simulink library "ControllerLibrary"  (R2016a)
settings: Solver=ode45  StartTime=0.0  StopTime=10.0  RelTol=1e-3
undefined symbols (not defined in the file or in its folder): ControlParams, ControlState, LegHipTorqueLimit, ps3Axes, ps3Buttons, ps3Pov, Ts
libraries: slrtlib x11, vrlib x1, simulink x1
settings Model: Creator=oharib  LastModifiedBy=oharib
settings DataIOCC: LimitDataPoints=on
settings DebuggingCC: AllowSymbolicDim=off

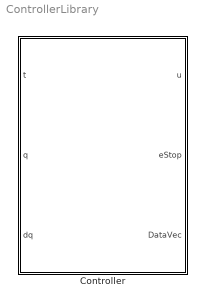
== system ControllerLibrary ==
  Controller : Subsystem

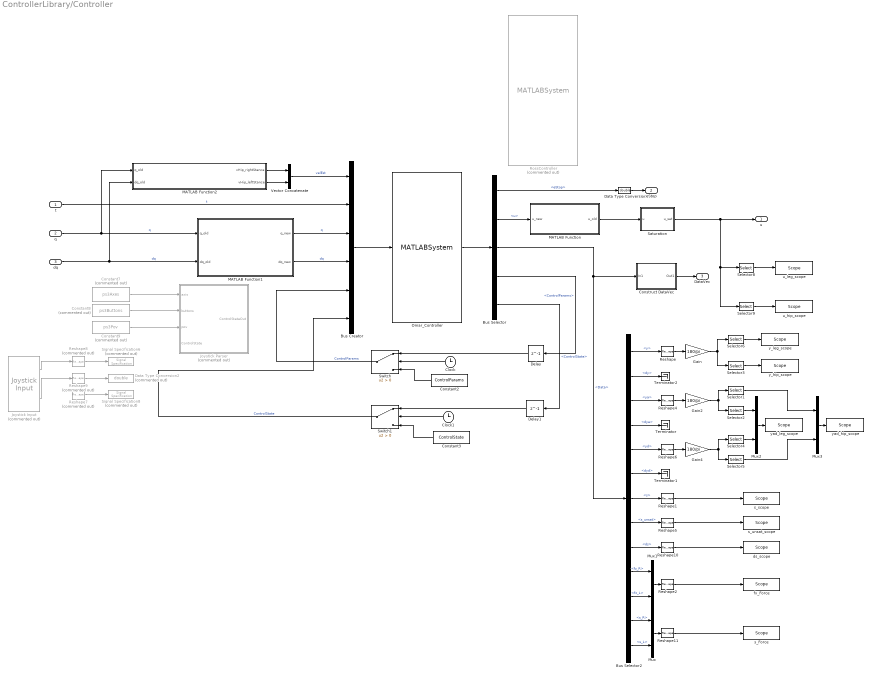
== system ControllerLibrary/Controller ==
  t : Inport
  q : Inport  Port=2
  dq : Inport  Port=3
  Bus Creator : BusCreator  Inputs='velEst','t','q','dq','ControlParams','ControlState'  OutDataTypeStr=Bus: Input_bus
  Bus Selector : BusSelector  OutputSignals=eStop,u,Data,ControlParams,ControlState
  Bus Selector2 : BusSelector  OutputSignals=y,dy,ya,dya,yd,dyd,s,s_unsat,ds,fz_R,fz_L,s_R,s_L
  Clock : Clock
  Clock1 : Clock
  Constant2 : Constant  Value=ControlParams  OutDataTypeStr=Bus: ControlParams_bus
  Constant3 : Constant  Value=ControlState  OutDataTypeStr=Bus: ControlState_bus
  Constant7 : Constant  Commented=on  Value=ps3Axes
  Constant8 : Constant  Commented=on  Value=ps3Buttons
  Constant9 : Constant  Commented=on  Value=ps3Pov
  Construct DataVec : Subsystem
  Data Type Conversion : DataTypeConversion  OutDataTypeStr=double
  Data Type Conversion2 : DataTypeConversion  Commented=on  OutDataTypeStr=double
  Delay : Delay  DelayLength=1  InitialCondition=0  InputProcessing=Inherited
  Delay1 : Delay  DelayLength=1  InitialCondition=0  InputProcessing=Inherited
  Gain : Gain  Gain=180/pi
  Gain2 : Gain  Gain=180/pi
  Gain4 : Gain  Gain=180/pi
  Joystick Input : vrlib/Joystick Input  Commented=on  joyid=1  adjustports=on  forcefeed=off
  Joystick Parser : Subsystem  Commented=on
  MATLAB Function : MATLAB Function  TreatAsAtomicUnit=on
  MATLAB Function1 : MATLAB Function  TreatAsAtomicUnit=on
  MATLAB Function2 : MATLAB Function  TreatAsAtomicUnit=on
  Mux{,1..3} (4 alike) : Mux  Inputs=2
  Omar_Controller : MATLABSystem  System=CompliantController.Omar_Controller  kp=kp_ctrl  kd=kd_ctrl  kp_hip=kp_hip_ctrl  kd_hip=kd_hip_ctrl  hold=hold_ctrl  shakeholdtest=1  controller_choice=controller_choice_ctrl  Ts=Ts  zero_error=zero_error_ctrl  torso_control=torso_control_ctrl  regulate_velocity=regulate_velocity_ctrl  threeD=threeD_ctrl  LimitSwHipAngle=LimitSwHipAngle_ctrl  jointPassivity=jointPassivity_ctrl  footPlacementLA=footPlacementLA_ctrl  footPlacementHA=footPlacementHA_ctrl  s_period=s_period_ctrl  number_of_domains_per_leg=4  deltaStKA=deltaStKA_ctrl  deltaSwKA=deltaSwKA_ctrl  deltaSwLA=deltaSwLA_ctrl  deltaSwHA=deltaSwHA_ctrl  joint_test_link_num=joint_test_link_num_ctrl  joint_test_freq=joint_test_freq_ctrl  joint_test_amp=joint_test_amp_ctrl  joint_zero=joint_zero_ctrl  isSim=isSim  OutputBusName=Output_bus  SimulateUsing=Code generation
      mask Type: CompliantController.Omar_Controller
      mask Display:
      | disp('Omar_Controller');
      | port_label('input',1,'input');
      | port_label('output',1,'output');
  Reshape{,1..2,4..6,10..11} (8 alike) : Reshape
  Reshape7 : Reshape  Commented=on  OutputDimensionality=Row vector (2-D)
  Reshape8 : Reshape  Commented=on  OutputDimensionality=Row vector (2-D)
  Reshape9 : Reshape  Commented=on  OutputDimensionality=Row vector (2-D)
  RossController : MATLABSystem  Commented=on  System=Ross_Controller_obj  kp_pitch=40  kd_pitch=1  kp_roll=40  kd_roll=1  kp_stanceLeg=40  kd_stanceLeg=1  kp_swingLeg=40  kd_swingLeg=1  kp_stanceKnee=40  kd_stanceKnee=1  kp_swingKnee=40  kd_swingKnee=1  kp_stanceHip=40  kd_stanceHip=1  kp_swingHip=40  kd_swingHip=1  tau=0.25  kf_sla=0  kp_sla=0.3  kd_sla=0.1  ki_sla=0  kg_sla=0  kf_sha=0.15  kp_sha=0.1  kd_sha=0.2  ki_sha=0  kg_sha=0  thres_lo=150  thres_hi=250  uHipGravity=0.9  springDeflectionImpactThreshold=0.0262  leg_length=0.6  torso_com_offset=[ 0; 0; 0 ]  isTest_holdInAir=false  isTest_doubleSupport=false  isTest_stopAndGo=false  isTest_constantHips=false  isTest_hipTracking=false  isSim=true  OutputBusName=Output_bus  SimulateUsing=Interpreted execution
      mask Type: Ross_Controller_obj
      mask Display:
      | disp('Ross_Controller_obj');
      | port_label('input',1,'input');
      | port_label('output',1,'output');
  Saturation : Subsystem
  Selector1 : Selector  InputPortWidth=6  IndexOptions=Index vector (dialog)  Indices=[1,4]  OutputSizes=1
  Selector2 : Selector  InputPortWidth=6  IndexOptions=Index vector (dialog)  Indices=[2,3,5,6]  OutputSizes=1
  Selector3 : Selector  InputPortWidth=6  IndexOptions=Index vector (dialog)  Indices=[1, 4]  OutputSizes=1
  Selector4 : Selector  InputPortWidth=6  IndexOptions=Index vector (dialog)  Indices=[2,3,5,6]  OutputSizes=1
  Selector5 : Selector  InputPortWidth=6  IndexOptions=Index vector (dialog)  Indices=[1,4]  OutputSizes=1
  Selector6 : Selector  InputPortWidth=6  IndexOptions=Index vector (dialog)  Indices=[2,3,5,6]  OutputSizes=1
  Selector8 : Selector  InputPortWidth=6  IndexOptions=Index vector (dialog)  Indices=[1, 2, 4, 5]  OutputSizes=1
  Selector9 : Selector  InputPortWidth=6  IndexOptions=Index vector (dialog)  Indices=[3, 6]  OutputSizes=1
  Signal Specification6 : SignalSpecification  Commented=on  OutDataTypeStr=double  Dimensions=5
  Signal Specification8 : SignalSpecification  Commented=on  OutDataTypeStr=double
  Switch : Switch  Criteria=u2 > Threshold
  Switch1 : Switch  Criteria=u2 > Threshold
  Terminator : Terminator
  Terminator1 : Terminator
  Terminator2 : Terminator
  Vector Concatenate : Concatenate
  ds_scope : slrtlib/Displays and Logging/Scope   scopeno=1  scopetype=Host  autostart=on  viewmode=Graphical redraw  formatstr='%15.6f'  grid=on  ylimits=[0,0]  nosamples=2500  noprepostsamples=0  interleave=1  triggermode=FreeRun  triggersignal=1  trigsignalfromport=off  triggerlevel=0.0  triggerslope=Either  triggerscope=1  triggersample=0  filename=data.dat  mode=Lazy  writesize=512  autorestart=off  dynamicfilemode=off  maxwritefilesize=512*1024^2
  fx_Force : slrtlib/Displays and Logging/Scope   scopeno=2  scopetype=Host  autostart=on  viewmode=Graphical redraw  formatstr='%15.6f'  grid=on  ylimits=[0,0]  nosamples=2500  noprepostsamples=0  interleave=1  triggermode=FreeRun  triggersignal=1  trigsignalfromport=off  triggerlevel=0.0  triggerslope=Either  triggerscope=1  triggersample=0  filename=data.dat  mode=Lazy  writesize=512  autorestart=off  dynamicfilemode=off  maxwritefilesize=512*1024^2
  s_Force : slrtlib/Displays and Logging/Scope   scopeno=14  scopetype=Host  autostart=on  viewmode=Graphical redraw  formatstr='%15.6f'  grid=on  ylimits=[0,0]  nosamples=2500  noprepostsamples=0  interleave=1  triggermode=FreeRun  triggersignal=1  trigsignalfromport=off  triggerlevel=0.0  triggerslope=Either  triggerscope=1  triggersample=0  filename=data.dat  mode=Lazy  writesize=512  autorestart=off  dynamicfilemode=off  maxwritefilesize=512*1024^2
  s_scope : slrtlib/Displays and Logging/Scope   scopeno=5  scopetype=Host  autostart=on  viewmode=Graphical redraw  formatstr='%15.6f'  grid=on  ylimits=[0,0]  nosamples=2500  noprepostsamples=0  interleave=1  triggermode=FreeRun  triggersignal=1  trigsignalfromport=off  triggerlevel=0.0  triggerslope=Either  triggerscope=1  triggersample=0  filename=data.dat  mode=Lazy  writesize=512  autorestart=off  dynamicfilemode=off  maxwritefilesize=512*1024^2
  s_unsat_scope : slrtlib/Displays and Logging/Scope   scopeno=6  scopetype=Host  autostart=on  viewmode=Graphical redraw  formatstr='%15.6f'  grid=on  ylimits=[0,0]  nosamples=2500  noprepostsamples=0  interleave=1  triggermode=FreeRun  triggersignal=1  trigsignalfromport=off  triggerlevel=0.0  triggerslope=Either  triggerscope=1  triggersample=0  filename=data.dat  mode=Lazy  writesize=512  autorestart=off  dynamicfilemode=off  maxwritefilesize=512*1024^2
  u_hip_scope : slrtlib/Displays and Logging/Scope   scopeno=8  scopetype=Host  autostart=on  viewmode=Graphical redraw  formatstr='%15.6f'  grid=on  ylimits=[0,0]  nosamples=2500  noprepostsamples=0  interleave=1  triggermode=FreeRun  triggersignal=1  trigsignalfromport=off  triggerlevel=0.0  triggerslope=Either  triggerscope=1  triggersample=0  filename=data.dat  mode=Lazy  writesize=512  autorestart=off  dynamicfilemode=off  maxwritefilesize=512*1024^2
  u_leg_scope : slrtlib/Displays and Logging/Scope   scopeno=7  scopetype=Host  autostart=on  viewmode=Graphical redraw  formatstr='%15.6f'  grid=on  ylimits=[0,0]  nosamples=2500  noprepostsamples=0  interleave=1  triggermode=FreeRun  triggersignal=1  trigsignalfromport=off  triggerlevel=0.0  triggerslope=Either  triggerscope=1  triggersample=0  filename=data.dat  mode=Lazy  writesize=512  autorestart=off  dynamicfilemode=off  maxwritefilesize=512*1024^2
  y_hip_scope : slrtlib/Displays and Logging/Scope   scopeno=9  scopetype=Host  autostart=on  viewmode=Graphical redraw  formatstr='%15.6f'  grid=on  ylimits=[0,0]  nosamples=2500  noprepostsamples=0  interleave=1  triggermode=FreeRun  triggersignal=1  trigsignalfromport=off  triggerlevel=0.0  triggerslope=Either  triggerscope=1  triggersample=0  filename=data.dat  mode=Lazy  writesize=512  autorestart=off  dynamicfilemode=off  maxwritefilesize=512*1024^2
  y_leg_scope : slrtlib/Displays and Logging/Scope   scopeno=4  scopetype=Host  autostart=on  viewmode=Graphical redraw  formatstr='%15.6f'  grid=on  ylimits=[0,0]  nosamples=2500  noprepostsamples=0  interleave=1  triggermode=FreeRun  triggersignal=1  trigsignalfromport=off  triggerlevel=0.0  triggerslope=Either  triggerscope=1  triggersample=0  filename=data.dat  mode=Lazy  writesize=512  autorestart=off  dynamicfilemode=off  maxwritefilesize=512*1024^2
  yad_hip_scope : slrtlib/Displays and Logging/Scope   scopeno=10  scopetype=Host  autostart=on  viewmode=Graphical redraw  formatstr='%15.6f'  grid=on  ylimits=[0,0]  nosamples=2500  noprepostsamples=0  interleave=1  triggermode=FreeRun  triggersignal=1  trigsignalfromport=off  triggerlevel=0.0  triggerslope=Either  triggerscope=1  triggersample=0  filename=data.dat  mode=Lazy  writesize=512  autorestart=off  dynamicfilemode=off  maxwritefilesize=512*1024^2
  yad_leg_scope : slrtlib/Displays and Logging/Scope   scopeno=3  scopetype=Host  autostart=on  viewmode=Graphical redraw  formatstr='%15.6f'  grid=on  ylimits=[0,0]  nosamples=2500  noprepostsamples=0  interleave=1  triggermode=FreeRun  triggersignal=1  trigsignalfromport=off  triggerlevel=0.0  triggerslope=Either  triggerscope=1  triggersample=0  filename=data.dat  mode=Lazy  writesize=512  autorestart=off  dynamicfilemode=off  maxwritefilesize=512*1024^2
  u : Outport  OutDataTypeStr=double
  eStop : Outport  Port=2  OutDataTypeStr=double
  DataVec : Outport  Port=3
  wires:
  dq/1 -> MATLAB Function2/2(dq_old), MATLAB Function1/2(dq_old)  "dq"
  Bus Selector/1 -> Data Type Conversion/1  "<eStop>"
  Data Type Conversion/1 -> eStop/1
  Saturation/1(u_sat) -> u/1, Selector8/1, Selector9/1
  t/1 -> Bus Creator/2  "t"
  Bus Creator/1 -> Omar_Controller/1
  Omar_Controller/1 -> Bus Selector/1
  Bus Selector/3 -> Bus Selector2/1, Construct DataVec/1(In1)  "<Data>"
  Bus Selector/4 -> Delay/1  "<ControlParams>"
  Bus Selector/5 -> Delay1/1  "<ControlState>"
  Delay/1 -> Switch/1
  Delay1/1 -> Switch1/1
  Clock/1 -> Switch/2
  Constant2/1 -> Switch/3
  Clock1/1 -> Switch1/2
  Constant3/1 -> Switch1/3
  Switch1/1 -> Bus Creator/6  "ControlState"
  Joystick Input/2 -> Reshape9/1
  Reshape8/1 -> Signal Specification6/1
  Joystick Input/1 -> Reshape8/1
  Reshape7/1 -> Signal Specification8/1
  Reshape9/1 -> Data Type Conversion2/1
  Construct DataVec/1(Out1) -> DataVec/1
  Constant7/1 -> Joystick Parser/1(axis)
  Constant8/1 -> Joystick Parser/2(buttons)
  q/1 -> MATLAB Function2/1(q_old), MATLAB Function1/1(q_old)  "q"
  MATLAB Function1/1(q_new) -> Bus Creator/3  "q"
  MATLAB Function/1(u_old) -> Saturation/1(u)
  Bus Selector/2 -> MATLAB Function/1(u_new)  "<u>"
  MATLAB Function1/2(dq_new) -> Bus Creator/4  "dq"
  Selector8/1 -> u_leg_scope/1
  Selector9/1 -> u_hip_scope/1
  Bus Selector2/1 -> Reshape/1  "<y>"
  Constant9/1 -> Joystick Parser/3(pov)
  Reshape/1 -> Gain/1
  Reshape4/1 -> Gain2/1
  Reshape6/1 -> Gain4/1
  Bus Selector2/5 -> Reshape6/1  "<yd>"
  Bus Selector2/3 -> Reshape4/1  "<ya>"
  Gain/1 -> Selector3/1, Selector6/1
  Selector3/1 -> y_hip_scope/1
  Bus Selector2/4 -> Terminator/1  "<dya>"
  Bus Selector2/6 -> Terminator1/1  "<dyd>"
  Bus Selector2/2 -> Terminator2/1  "<dy>"
  MATLAB Function2/1(vHip_rightStance) -> Vector Concatenate/1
  MATLAB Function2/2(vHip_leftStance) -> Vector Concatenate/2
  Vector Concatenate/1 -> Bus Creator/1  "velEst"
  Bus Selector2/9 -> Reshape10/1  "<ds>"
  Reshape10/1 -> ds_scope/1
  Reshape5/1 -> s_unsat_scope/1
  Reshape1/1 -> s_scope/1
  Bus Selector2/7 -> Reshape1/1  "<s>"
  Bus Selector2/8 -> Reshape5/1  "<s_unsat>"
  Reshape11/1 -> s_Force/1
  Bus Selector2/12 -> Mux/1  "<s_R>"
  Bus Selector2/13 -> Mux/2  "<s_L>"
  Mux/1 -> Reshape11/1
  Reshape2/1 -> fx_Force/1
  Bus Selector2/10 -> Mux1/1  "<fz_R>"
  Bus Selector2/11 -> Mux1/2  "<fz_L>"
  Mux1/1 -> Reshape2/1
  Gain2/1 -> Selector1/1, Selector2/1
  Gain4/1 -> Selector5/1, Selector4/1
  Selector6/1 -> y_leg_scope/1
  Mux2/1 -> yad_leg_scope/1
  Selector2/1 -> Mux2/1
  Selector4/1 -> Mux2/2
  Mux3/1 -> yad_hip_scope/1
  Selector1/1 -> Mux3/1
  Selector5/1 -> Mux3/2
  Switch/1 -> Bus Creator/5  "ControlParams"

== system ControllerLibrary/Controller/Construct DataVec ==
  In1 : Inport
  DataBusSelector : BusSelector  OutputSignals=q,u,y,dy,ya,dya,yd,dyd,s,s_unsat,ds,Domain,s_R,s_L,fz_R,fz_L,velFiltered,velMeasured,swingHipAdjustment,swingLegAdjustment
  DataVectorize : Concatenate  NumInputs=20
  Out1 : Outport
  wires:
  In1/1 -> DataBusSelector/1
  DataVectorize/1 -> Out1/1
  DataBusSelector/1 -> DataVectorize/1  "<q>"
  DataBusSelector/2 -> DataVectorize/2  "<u>"
  DataBusSelector/3 -> DataVectorize/3  "<y>"
  DataBusSelector/4 -> DataVectorize/4  "<dy>"
  DataBusSelector/5 -> DataVectorize/5  "<ya>"
  DataBusSelector/6 -> DataVectorize/6  "<dya>"
  DataBusSelector/7 -> DataVectorize/7  "<yd>"
  DataBusSelector/8 -> DataVectorize/8  "<dyd>"
  DataBusSelector/9 -> DataVectorize/9  "<s>"
  DataBusSelector/10 -> DataVectorize/10  "<s_unsat>"
  DataBusSelector/11 -> DataVectorize/11  "<ds>"
  DataBusSelector/12 -> DataVectorize/12  "<Domain>"
  DataBusSelector/13 -> DataVectorize/13  "<s_R>"
  DataBusSelector/14 -> DataVectorize/14  "<s_L>"
  DataBusSelector/15 -> DataVectorize/15  "<fz_R>"
  DataBusSelector/16 -> DataVectorize/16  "<fz_L>"
  DataBusSelector/17 -> DataVectorize/17  "<velFiltered>"
  DataBusSelector/18 -> DataVectorize/18  "<velMeasured>"
  DataBusSelector/19 -> DataVectorize/19  "<swingHipAdjustment>"
  DataBusSelector/20 -> DataVectorize/20  "<swingLegAdjustment>"

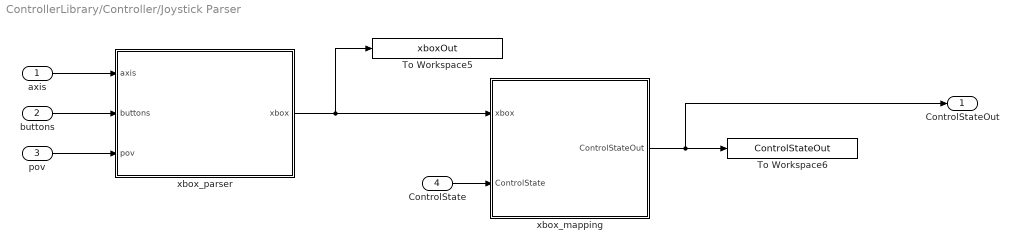
== system ControllerLibrary/Controller/Joystick Parser ==
  axis : Inport
  buttons : Inport  Port=2
  pov : Inport  Port=3
  ControlState : Inport  Port=4  OutDataTypeStr=Bus: ControlState_bus
  To Workspace5 : ToWorkspace  VariableName=xboxOut  SaveFormat=Timeseries  SampleTime=-1
  To Workspace6 : ToWorkspace  VariableName=ControlStateOut  SaveFormat=Timeseries  SampleTime=-1
  xbox_mapping : Subsystem
  xbox_parser : MATLAB Function  TreatAsAtomicUnit=on
  ControlStateOut : Outport  OutDataTypeStr=Bus: ControlState_bus
  wires:
  xbox_parser/1(xbox) -> To Workspace5/1, xbox_mapping/1(xbox)
  xbox_mapping/1(ControlStateOut) -> To Workspace6/1, ControlStateOut/1
  axis/1 -> xbox_parser/1(axis)
  buttons/1 -> xbox_parser/2(buttons)
  pov/1 -> xbox_parser/3(pov)
  ControlState/1 -> xbox_mapping/2(ControlState)

== system ControllerLibrary/Controller/Saturation ==
  u : Inport
  Data Type Conversion1 : DataTypeConversion  OutDataTypeStr=double
  Gain : Gain  Gain=-1
  Gain1 : Gain  Gain=[1 0; 1 0; 0 1; 1 0; 1 0; 0 1]  Multiplication=Matrix(K*u)
  LegHipTorqueSat : Constant  Value=LegHipTorqueLimit
  Saturation Dynamic : simulink/Discontinuities/Saturation Dynamic  OutMin=[]  OutMax=[]  OutDataTypeStr=Inherit: Same as second input  OutDataType=fixdt(1, 16)  OutScaling=2^-10  DoSatur=off
  u_sat : Outport  OutDataTypeStr=double
  wires:
  Saturation Dynamic/1 -> Data Type Conversion1/1
  Data Type Conversion1/1 -> u_sat/1  "torque_sat"
  LegHipTorqueSat/1 -> Gain1/1
  Gain1/1 -> Saturation Dynamic/1, Gain/1
  Gain/1 -> Saturation Dynamic/3
  u/1 -> Saturation Dynamic/2

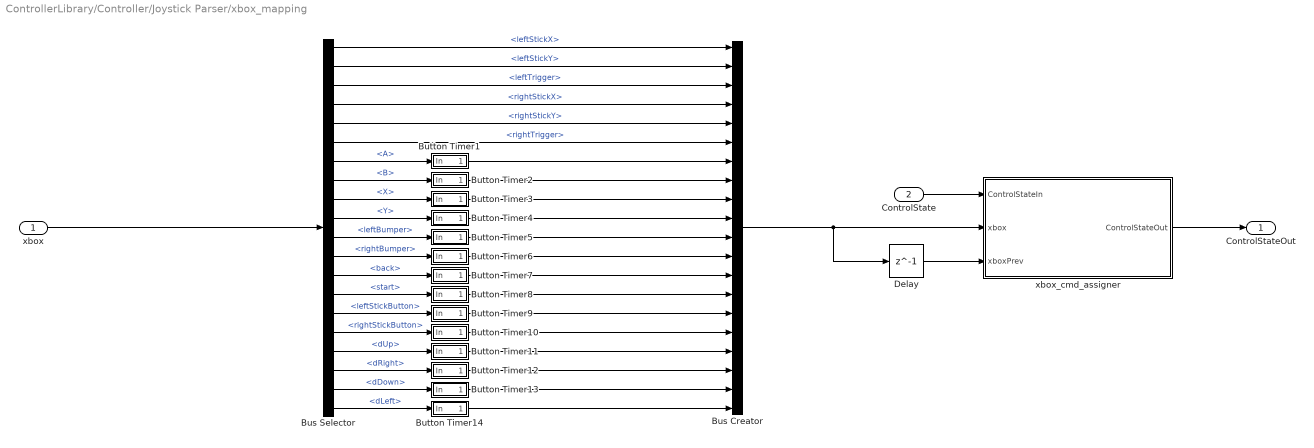
== system ControllerLibrary/Controller/Joystick Parser/xbox_mapping ==
  xbox : Inport
  ControlState : Inport  Port=2  OutDataTypeStr=Bus: ControlState_bus
  Bus Creator : BusCreator  Inputs=20  OutDataTypeStr=Bus: xbox_bus  NonVirtualBus=on
  Bus Selector : BusSelector  OutputSignals=leftStickX,leftStickY,leftTrigger,rightStickX,rightStickY,rightTrigger,A,B,X,Y,leftBumper,rightBumper,back,start,leftStickButton,rightStickButton,dUp,dRight,dDown,dLeft
  Button Timer1 : Subsystem
  Button Timer10 : Subsystem
  Button Timer11 : Subsystem
  Button Timer12 : Subsystem
  Button Timer13 : Subsystem
  Button Timer14 : Subsystem
  Button Timer2 : Subsystem
  Button Timer3 : Subsystem
  Button Timer4 : Subsystem
  Button Timer5 : Subsystem
  Button Timer6 : Subsystem
  Button Timer7 : Subsystem
  Button Timer8 : Subsystem
  Button Timer9 : Subsystem
  Delay : Delay  DelayLength=1  InitialCondition=0
  xbox_cmd_assigner : MATLAB Function  TreatAsAtomicUnit=on
  ControlStateOut : Outport  OutDataTypeStr=Bus: ControlState_bus
  wires:
  Bus Selector/12 -> Button Timer6/1(In)  "<rightBumper>"
  Bus Selector/4 -> Bus Creator/4  "<rightStickX>"
  Bus Selector/3 -> Bus Creator/3  "<leftTrigger>"
  Bus Selector/9 -> Button Timer3/1(In)  "<X>"
  Bus Selector/1 -> Bus Creator/1  "<leftStickX>"
  Bus Selector/5 -> Bus Creator/5  "<rightStickY>"
  Bus Selector/14 -> Button Timer8/1(In)  "<start>"
  Bus Selector/17 -> Button Timer11/1(In)  "<dUp>"
  Bus Selector/18 -> Button Timer12/1(In)  "<dRight>"
  Bus Selector/8 -> Button Timer2/1(In)  "<B>"
  Bus Selector/19 -> Button Timer13/1(In)  "<dDown>"
  Bus Selector/7 -> Button Timer1/1(In)  "<A>"
  Bus Selector/15 -> Button Timer9/1(In)  "<leftStickButton>"
  xbox/1 -> Bus Selector/1
  Bus Selector/6 -> Bus Creator/6  "<rightTrigger>"
  Bus Selector/20 -> Button Timer14/1(In)  "<dLeft>"
  Bus Selector/2 -> Bus Creator/2  "<leftStickY>"
  Bus Selector/10 -> Button Timer4/1(In)  "<Y>"
  Bus Selector/13 -> Button Timer7/1(In)  "<back>"
  Bus Selector/16 -> Button Timer10/1(In)  "<rightStickButton>"
  Bus Selector/11 -> Button Timer5/1(In)  "<leftBumper>"
  Button Timer2/1(Out) -> Bus Creator/8
  Button Timer4/1(Out) -> Bus Creator/10
  Button Timer5/1(Out) -> Bus Creator/11
  Button Timer6/1(Out) -> Bus Creator/12
  Button Timer7/1(Out) -> Bus Creator/13
  Button Timer8/1(Out) -> Bus Creator/14
  Button Timer9/1(Out) -> Bus Creator/15
  Button Timer10/1(Out) -> Bus Creator/16
  Button Timer11/1(Out) -> Bus Creator/17
  Button Timer12/1(Out) -> Bus Creator/18
  Button Timer13/1(Out) -> Bus Creator/19
  Button Timer14/1(Out) -> Bus Creator/20
  Bus Creator/1 -> Delay/1, xbox_cmd_assigner/2(xbox)
  ControlState/1 -> xbox_cmd_assigner/1(ControlStateIn)
  Button Timer1/1(Out) -> Bus Creator/7
  Button Timer3/1(Out) -> Bus Creator/9
  xbox_cmd_assigner/1(ControlStateOut) -> ControlStateOut/1
  Delay/1 -> xbox_cmd_assigner/3(xboxPrev)

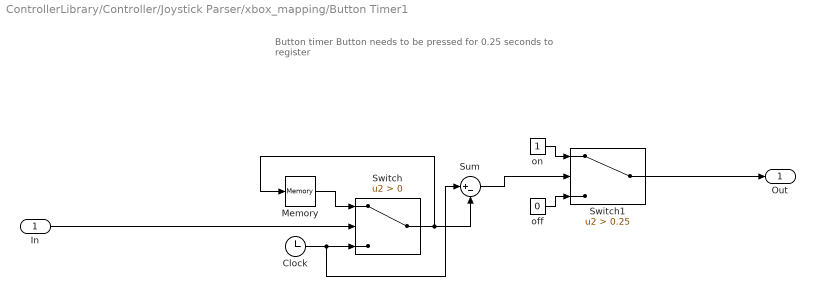
== system ControllerLibrary/Controller/Joystick Parser/xbox_mapping/Button Timer1 ==
  note: Button timer
      | Button needs to be pressed for 0.25 seconds to register
  In : Inport
  Clock : Clock
  Memory : Memory
  Sum : Sum  Inputs=|+-
  Switch : Switch  Criteria=u2 > Threshold
  Switch1 : Switch  Criteria=u2 > Threshold  Threshold=0.25
  off : Constant  Value=0
  on : Constant
  Out : Outport
  wires:
  off/1 -> Switch1/3
  Sum/1 -> Switch1/2
  Switch1/1 -> Out/1
  on/1 -> Switch1/1
  In/1 -> Switch/2
  Clock/1 -> Sum/1, Switch/3
  Memory/1 -> Switch/1
  Switch/1 -> Sum/2, Memory/1

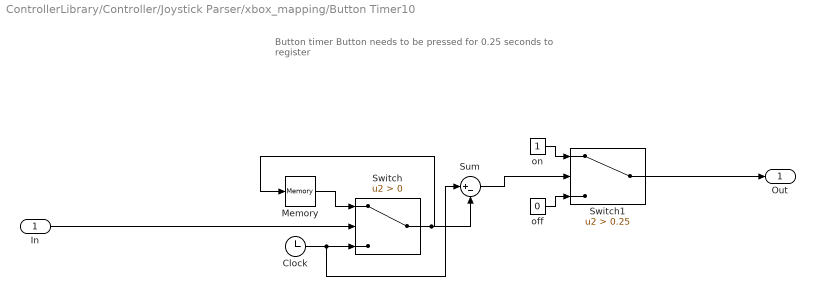
== system ControllerLibrary/Controller/Joystick Parser/xbox_mapping/Button Timer10 ==
  note: Button timer
      | Button needs to be pressed for 0.25 seconds to register
  In : Inport
  Clock : Clock
  Memory : Memory
  Sum : Sum  Inputs=|+-
  Switch : Switch  Criteria=u2 > Threshold
  Switch1 : Switch  Criteria=u2 > Threshold  Threshold=0.25
  off : Constant  Value=0
  on : Constant
  Out : Outport
  wires:
  off/1 -> Switch1/3
  Sum/1 -> Switch1/2
  Switch1/1 -> Out/1
  on/1 -> Switch1/1
  In/1 -> Switch/2
  Clock/1 -> Sum/1, Switch/3
  Memory/1 -> Switch/1
  Switch/1 -> Sum/2, Memory/1

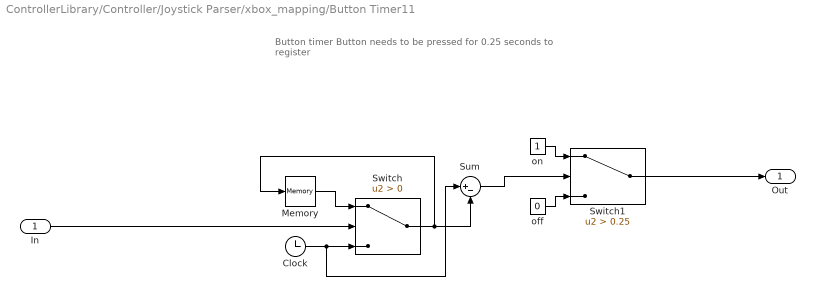
== system ControllerLibrary/Controller/Joystick Parser/xbox_mapping/Button Timer11 ==
  note: Button timer
      | Button needs to be pressed for 0.25 seconds to register
  In : Inport
  Clock : Clock
  Memory : Memory
  Sum : Sum  Inputs=|+-
  Switch : Switch  Criteria=u2 > Threshold
  Switch1 : Switch  Criteria=u2 > Threshold  Threshold=0.25
  off : Constant  Value=0
  on : Constant
  Out : Outport
  wires:
  off/1 -> Switch1/3
  Sum/1 -> Switch1/2
  Switch1/1 -> Out/1
  on/1 -> Switch1/1
  In/1 -> Switch/2
  Clock/1 -> Sum/1, Switch/3
  Memory/1 -> Switch/1
  Switch/1 -> Sum/2, Memory/1

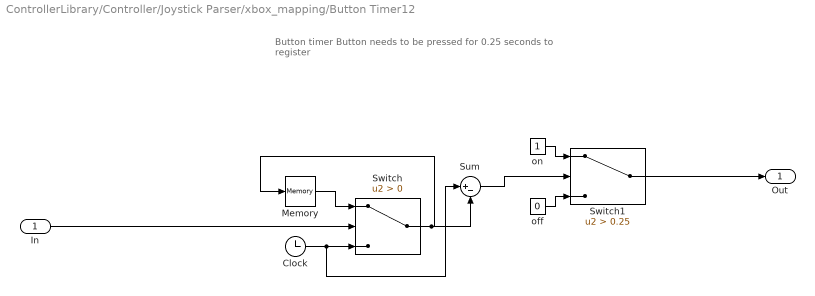
== system ControllerLibrary/Controller/Joystick Parser/xbox_mapping/Button Timer12 ==
  note: Button timer
      | Button needs to be pressed for 0.25 seconds to register
  In : Inport
  Clock : Clock
  Memory : Memory
  Sum : Sum  Inputs=|+-
  Switch : Switch  Criteria=u2 > Threshold
  Switch1 : Switch  Criteria=u2 > Threshold  Threshold=0.25
  off : Constant  Value=0
  on : Constant
  Out : Outport
  wires:
  off/1 -> Switch1/3
  Sum/1 -> Switch1/2
  Switch1/1 -> Out/1
  on/1 -> Switch1/1
  In/1 -> Switch/2
  Clock/1 -> Sum/1, Switch/3
  Memory/1 -> Switch/1
  Switch/1 -> Sum/2, Memory/1

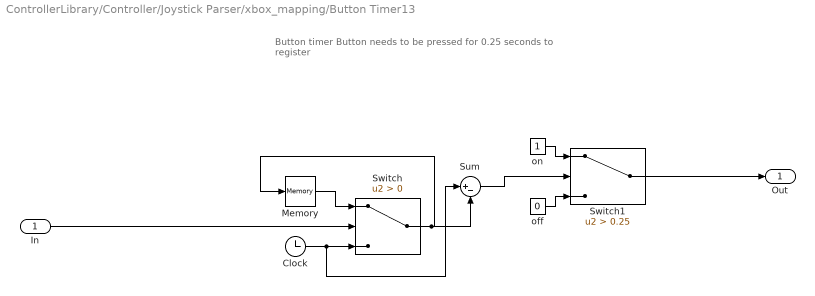
== system ControllerLibrary/Controller/Joystick Parser/xbox_mapping/Button Timer13 ==
  note: Button timer
      | Button needs to be pressed for 0.25 seconds to register
  In : Inport
  Clock : Clock
  Memory : Memory
  Sum : Sum  Inputs=|+-
  Switch : Switch  Criteria=u2 > Threshold
  Switch1 : Switch  Criteria=u2 > Threshold  Threshold=0.25
  off : Constant  Value=0
  on : Constant
  Out : Outport
  wires:
  off/1 -> Switch1/3
  Sum/1 -> Switch1/2
  Switch1/1 -> Out/1
  on/1 -> Switch1/1
  In/1 -> Switch/2
  Clock/1 -> Sum/1, Switch/3
  Memory/1 -> Switch/1
  Switch/1 -> Sum/2, Memory/1

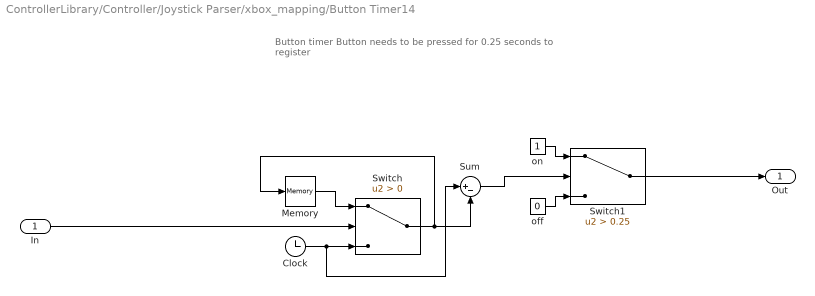
== system ControllerLibrary/Controller/Joystick Parser/xbox_mapping/Button Timer14 ==
  note: Button timer
      | Button needs to be pressed for 0.25 seconds to register
  In : Inport
  Clock : Clock
  Memory : Memory
  Sum : Sum  Inputs=|+-
  Switch : Switch  Criteria=u2 > Threshold
  Switch1 : Switch  Criteria=u2 > Threshold  Threshold=0.25
  off : Constant  Value=0
  on : Constant
  Out : Outport
  wires:
  off/1 -> Switch1/3
  Sum/1 -> Switch1/2
  Switch1/1 -> Out/1
  on/1 -> Switch1/1
  In/1 -> Switch/2
  Clock/1 -> Sum/1, Switch/3
  Memory/1 -> Switch/1
  Switch/1 -> Sum/2, Memory/1

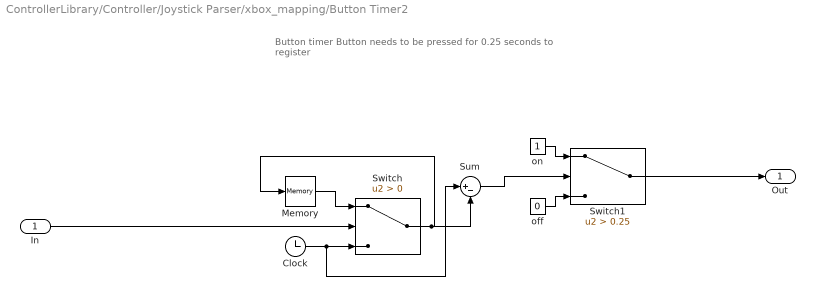
== system ControllerLibrary/Controller/Joystick Parser/xbox_mapping/Button Timer2 ==
  note: Button timer
      | Button needs to be pressed for 0.25 seconds to register
  In : Inport
  Clock : Clock
  Memory : Memory
  Sum : Sum  Inputs=|+-
  Switch : Switch  Criteria=u2 > Threshold
  Switch1 : Switch  Criteria=u2 > Threshold  Threshold=0.25
  off : Constant  Value=0
  on : Constant
  Out : Outport
  wires:
  off/1 -> Switch1/3
  Sum/1 -> Switch1/2
  Switch1/1 -> Out/1
  on/1 -> Switch1/1
  In/1 -> Switch/2
  Clock/1 -> Sum/1, Switch/3
  Memory/1 -> Switch/1
  Switch/1 -> Sum/2, Memory/1

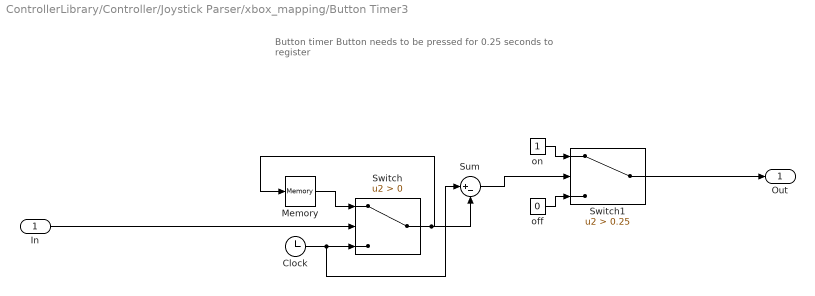
== system ControllerLibrary/Controller/Joystick Parser/xbox_mapping/Button Timer3 ==
  note: Button timer
      | Button needs to be pressed for 0.25 seconds to register
  In : Inport
  Clock : Clock
  Memory : Memory
  Sum : Sum  Inputs=|+-
  Switch : Switch  Criteria=u2 > Threshold
  Switch1 : Switch  Criteria=u2 > Threshold  Threshold=0.25
  off : Constant  Value=0
  on : Constant
  Out : Outport
  wires:
  off/1 -> Switch1/3
  Sum/1 -> Switch1/2
  Switch1/1 -> Out/1
  on/1 -> Switch1/1
  In/1 -> Switch/2
  Clock/1 -> Sum/1, Switch/3
  Memory/1 -> Switch/1
  Switch/1 -> Sum/2, Memory/1

== system ControllerLibrary/Controller/Joystick Parser/xbox_mapping/Button Timer4 ==
  note: Button timer
      | Button needs to be pressed for 0.25 seconds to register
  In : Inport
  Clock : Clock
  Memory : Memory
  Sum : Sum  Inputs=|+-
  Switch : Switch  Criteria=u2 > Threshold
  Switch1 : Switch  Criteria=u2 > Threshold  Threshold=0.25
  off : Constant  Value=0
  on : Constant
  Out : Outport
  wires:
  off/1 -> Switch1/3
  Sum/1 -> Switch1/2
  Switch1/1 -> Out/1
  on/1 -> Switch1/1
  In/1 -> Switch/2
  Clock/1 -> Sum/1, Switch/3
  Memory/1 -> Switch/1
  Switch/1 -> Sum/2, Memory/1

== system ControllerLibrary/Controller/Joystick Parser/xbox_mapping/Button Timer5 ==
  note: Button timer
      | Button needs to be pressed for 0.25 seconds to register
  In : Inport
  Clock : Clock
  Memory : Memory
  Sum : Sum  Inputs=|+-
  Switch : Switch  Criteria=u2 > Threshold
  Switch1 : Switch  Criteria=u2 > Threshold  Threshold=0.25
  off : Constant  Value=0
  on : Constant
  Out : Outport
  wires:
  off/1 -> Switch1/3
  Sum/1 -> Switch1/2
  Switch1/1 -> Out/1
  on/1 -> Switch1/1
  In/1 -> Switch/2
  Clock/1 -> Sum/1, Switch/3
  Memory/1 -> Switch/1
  Switch/1 -> Sum/2, Memory/1

== system ControllerLibrary/Controller/Joystick Parser/xbox_mapping/Button Timer6 ==
  note: Button timer
      | Button needs to be pressed for 0.25 seconds to register
  In : Inport
  Clock : Clock
  Memory : Memory
  Sum : Sum  Inputs=|+-
  Switch : Switch  Criteria=u2 > Threshold
  Switch1 : Switch  Criteria=u2 > Threshold  Threshold=0.25
  off : Constant  Value=0
  on : Constant
  Out : Outport
  wires:
  off/1 -> Switch1/3
  Sum/1 -> Switch1/2
  Switch1/1 -> Out/1
  on/1 -> Switch1/1
  In/1 -> Switch/2
  Clock/1 -> Sum/1, Switch/3
  Memory/1 -> Switch/1
  Switch/1 -> Sum/2, Memory/1

== system ControllerLibrary/Controller/Joystick Parser/xbox_mapping/Button Timer7 ==
  note: Button timer
      | Button needs to be pressed for 0.25 seconds to register
  In : Inport
  Clock : Clock
  Memory : Memory
  Sum : Sum  Inputs=|+-
  Switch : Switch  Criteria=u2 > Threshold
  Switch1 : Switch  Criteria=u2 > Threshold  Threshold=0.25
  off : Constant  Value=0
  on : Constant
  Out : Outport
  wires:
  off/1 -> Switch1/3
  Sum/1 -> Switch1/2
  Switch1/1 -> Out/1
  on/1 -> Switch1/1
  In/1 -> Switch/2
  Clock/1 -> Sum/1, Switch/3
  Memory/1 -> Switch/1
  Switch/1 -> Sum/2, Memory/1

== system ControllerLibrary/Controller/Joystick Parser/xbox_mapping/Button Timer8 ==
  note: Button timer
      | Button needs to be pressed for 0.25 seconds to register
  In : Inport
  Clock : Clock
  Memory : Memory
  Sum : Sum  Inputs=|+-
  Switch : Switch  Criteria=u2 > Threshold
  Switch1 : Switch  Criteria=u2 > Threshold  Threshold=0.25
  off : Constant  Value=0
  on : Constant
  Out : Outport
  wires:
  off/1 -> Switch1/3
  Sum/1 -> Switch1/2
  Switch1/1 -> Out/1
  on/1 -> Switch1/1
  In/1 -> Switch/2
  Clock/1 -> Sum/1, Switch/3
  Memory/1 -> Switch/1
  Switch/1 -> Sum/2, Memory/1

== system ControllerLibrary/Controller/Joystick Parser/xbox_mapping/Button Timer9 ==
  note: Button timer
      | Button needs to be pressed for 0.25 seconds to register
  In : Inport
  Clock : Clock
  Memory : Memory
  Sum : Sum  Inputs=|+-
  Switch : Switch  Criteria=u2 > Threshold
  Switch1 : Switch  Criteria=u2 > Threshold  Threshold=0.25
  off : Constant  Value=0
  on : Constant
  Out : Outport
  wires:
  off/1 -> Switch1/3
  Sum/1 -> Switch1/2
  Switch1/1 -> Out/1
  on/1 -> Switch1/1
  In/1 -> Switch/2
  Clock/1 -> Sum/1, Switch/3
  Memory/1 -> Switch/1
  Switch/1 -> Sum/2, Memory/1

== matlab function ControllerLibrary/Controller/MATLAB Function ==
  data: u_new input; u_old output
function u_old = Convert_u_to_old_coordinates(u_new)
%#codegen

% u_new = [qHR, qAR, qBR, qHL, qAL, qBL]
% u_old = [qAR, qBR, qHR, qAL, qBL, qHL]

u_old = u_new([2,3,1,5,6,4]);
u_old(6) = -u_old(6); % Flip left hip torque

end

== matlab function ControllerLibrary/Controller/MATLAB Function1 ==
  data: q_old input; q_new output; dq_old input; dq_new output
function [q_new, dq_new] = Convert_x_to_new_coordinates(q_old, dq_old)
%#codegen
[q_new, dq_new] = CompliantSystem.ConvertToNewCoord(q_old, dq_old);
end

== matlab function ControllerLibrary/Controller/Joystick Parser/xbox_mapping/xbox_cmd_assigner ==
  data: ControlStateIn input; xbox input; ControlStateOut output Bus: ControlState_bus; xboxPrev input
function ControlStateOut = xbox_cmd_assigner(ControlStateIn, xbox, xboxPrev) %#codegen
%% Copyright 2016 - Ross Hartley

ControlStateOut = ControlStateIn;
sampleInterval = 0.0005;

%% Commands 

% Shutdown
if xbox.back == 1
	ControlStateOut.Commands.Shutdown = 1;
end

% Enable
if xbox.start == 1
	ControlStateOut.Commands.EnableTransition = 1;
end

% If rightBumper is pressed, reset state estimator
if (xbox.rightBumper == 1) && (xboxPrev.rightBumper == 0) % Rising edge
	ControlStateOut.Commands.ResetStateEstimator = 1;
else
    ControlStateOut.Commands.ResetStateEstimator = 0;
end

% If leftBumper is pressed, calibrate offsets
if (xbox.leftBumper == 1) && (xboxPrev.leftBumper == 0) % Rising edge
    ControlStateOut.Commands.IntegralControl = ~ControlStateOut.Commands.IntegralControl;
end

% Parse right joystick for time scaling tests
TimeScale = max(min(xbox.rightStickY, 1), -1);
alpha_ts = sampleInterval/(2 + sampleInterval);
ControlStateOut.Commands.TimeScale = ControlStateOut.Commands.TimeScale + alpha_ts*(TimeScale - ControlStateOut.Commands.TimeScale);
% If rightBumper is pressed, pause time
if (xbox.rightBumper == 1) && (xboxPrev.rightBumper == 0) % Rising edge
    ControlStateOut.Commands.PauseTime = ~ControlStateOut.Commands.PauseTime;
end
    
if ControlStateIn.Options.Enable_dy_tgt
    % Parse left joystick data for Y Velocity
    dy_cmd = max(min(xbox.leftStickY, 0.8), -0.8);
    if abs(dy_cmd) < 0.1
        dy_cmd = 0; % Ignore small values
    end
    % Filter target X velocity command
    alpha_dy = sampleInterval/(2 + sampleInterval);
    ControlStateOut.Commands.dy_tgt = ControlStateOut.Commands.dy_tgt + alpha_dy*(dy_cmd - ControlStateOut.Commands.dy_tgt);
end

if ControlStateIn.Options.Enable_dx_tgt
    % Parse right joystick data for X Velocity
    dx_cmd = max(min(xbox.rightStickX, 0.5), -0.5);
    if abs(dx_cmd) < 0.1
        dx_cmd = 0; % Ignore small values
    end
    % Filter target X velocity command
    alpha_dx = sampleInterval/(2 + sampleInterval);
    ControlStateOut.Commands.dx_tgt = ControlStateOut.Commands.dx_tgt + alpha_dx*(dx_cmd - ControlStateOut.Commands.dx_tgt);
end

% Activate Side Stepping
if xbox.X == 1 && ControlStateIn.Options.EnableSideStep
	ControlStateOut.Commands.ActivateSideStepLeft = 1;
else
	ControlStateOut.Commands.ActivateSideStepLeft = 0;
end

% Activate Kicking
if xbox.A == 1 && ControlStateIn.Options.EnableKicking
	ControlStateOut.Commands.ActivateKickingLeft = 1;
else
	ControlStateOut.Commands.ActivateKickingLeft = 0;
end

%% Offsets

% Center of Mass offsets
if (xbox.dUp == 1) && (xboxPrev.dUp == 0) % Rising edge
	ControlStateOut.Offsets.yOffset = ControlStateOut.Offsets.yOffset + 0.001;
end
if (xbox.dDown == 1) && (xboxPrev.dDown == 0) % Rising edge
	ControlStateOut.Offsets.yOffset = ControlStateOut.Offsets.yOffset - 0.001;
end
if (xbox.dRight == 1) && (xboxPrev.dRight == 0) % Rising edge
	ControlStateOut.Offsets.xOffset = ControlStateOut.Offsets.xOffset + 0.001;
end
if (xbox.dLeft == 1) && (xboxPrev.dLeft == 0) % Rising edge
	ControlStateOut.Offsets.xOffset = ControlStateOut.Offsets.xOffset - 0.001;
end


end

== matlab function ControllerLibrary/Controller/Joystick Parser/xbox_parser ==
  data: axis input; xbox output Bus: xbox_bus; buttons input; pov input
function xbox = xbox_parser(axis, buttons, pov)
%#codegen

% axis parsing
xbox.leftStickX = axis(1);
xbox.leftStickY = -axis(2);
xbox.leftTrigger = axis(3);
xbox.rightStickX = axis(4);
xbox.rightStickY = -axis(5);
%xbox.rightTrigger = axis(6);
xbox.rightTrigger = axis(3);

% button parsing
xbox.A = buttons(1);
xbox.B = buttons(2);
xbox.X = buttons(3);
xbox.Y = buttons(4);
xbox.leftBumper = buttons(5);
xbox.rightBumper = buttons(6);
xbox.back = buttons(7);
xbox.start = buttons(8);
xbox.leftStickButton = buttons(9);
xbox.rightStickButton = buttons(10);

% D-pad parsing
switch pov
	case -1
		xbox.dUp = 0;
		xbox.dRight = 0;
		xbox.dDown = 0;
		xbox.dLeft = 0;
		
	case 0
		xbox.dUp = 1;
		xbox.dRight = 0;
		xbox.dDown = 0;
		xbox.dLeft = 0;
		
	case 45
		xbox.dUp = 1;
		xbox.dRight = 1;
		xbox.dDown = 0;
		xbox.dLeft = 0;
		
	case 90
		xbox.dUp = 0;
		xbox.dRight = 1;
		xbox.dDown = 0;
		xbox.dLeft = 0;
		
	case 135
		xbox.dUp = 0;
		xbox.dRight = 1;
		xbox.dDown = 1;
		xbox.dLeft = 0;
		
	case 180
		xbox.dUp = 0;
		xbox.dRight = 0;
		xbox.dDown = 1;
		xbox.dLeft = 0;
		
	case 225
		xbox.dUp = 0;
		xbox.dRight = 0;
		xbox.dDown = 1;
		xbox.dLeft = 1;
	
	case 270
		xbox.dUp = 0;
		xbox.dRight = 0;
		xbox.dDown = 0;
		xbox.dLeft = 1;
		
	case 315
		xbox.dUp = 1;
		xbox.dRight = 0;
		xbox.dDown = 0;
		xbox.dLeft = 1;
		
	otherwise
		xbox.dUp = 0;
		xbox.dRight = 0;
		xbox.dDown = 0;
		xbox.dLeft = 0;
		
end
		
end

== matlab function ControllerLibrary/Controller/MATLAB Function2 ==
  data: q_old input; vHip_rightStance output; dq_old input; vHip_leftStance output
function [vHip_rightStance, vHip_leftStance] = EstimateVelocity_Kinematics(q_old, dq_old)
q = q_old;
dq = dq_old;

% Leg Length (L4)
leg_length = 0.6;
torso_com_offset = [0;0;0];

[~, ~, ~, ~, ~, ~, vHip_rightStance] = OriginalLeg_Springs_VariableLeg_COMoffset.ATRIAS3D_VelocitiesAccel_Right([0;q(2:end)], dq, [leg_length;torso_com_offset]);
[~, ~, ~, ~, ~, ~, vHip_leftStance] = OriginalLeg_Springs_VariableLeg_COMoffset.ATRIAS3D_VelocitiesAccel_Left([0;q(2:end)], dq, [leg_length;torso_com_offset]);
end
